simulink model "daqp_block"  (Simulink 10.3)
settings: Solver=VariableStepAuto  StartTime=0.0  StopTime=10.0  RelTol=1e-3
settings Model: Creator=danar20  LastModifiedBy=danar20
settings SolverCC: AlgebraicLoopSolver=Auto
settings DataIOCC: SaveFormat=Dataset  SignalLoggingSaveFormat=Dataset  ReturnWorkspaceOutputs=on
settings OptimizationCC: ExpressionDepthLimit=128  LifeSpan=auto
settings DebuggingCC: UnderspecifiedInitializationDetection=Simplified  MergeDetectMultiDrivingBlocksExec=error  FcnCallInpInsideContextMsg=error  StateNameClashWarn=none  SFUnexpectedBacktrackingDiag=error  SFNoUnconditionalDefaultTransitionDiag=error  SFExecutionAtInitializationDiag=warning  SFMachineParentedDataDiag=error  ArithmeticOperatorsInVariantConditions=error
settings HardwareCC: ProdBitPerPointer=64  ProdBitPerSizeT=64  ProdBitPerPtrDiffT=64  ProdLargestAtomicFloat=Float  ProdIntDivRoundTo=Zero  ProdEndianess=LittleEndian  ProdWordSize=64  ProdHWDeviceType=Intel->x86-64 (Windows64)
settings ModelReferenceCC: PropagateSignalLabelsOutOfModel=on
settings SFSimCC: SimUseLocalCustomCode=on  CustomCodeUndefinedFunction=FilterOut
settings RTWCC: RTWUseLocalCustomCode=on
settings CodeAppCC: StateflowObjectComments=off
settings GRTTargetCC: TargetLangStandard=C99 (ISO)  CombineOutputUpdateFcns=on  GRTInterface=off
settings ConfigComp: CovMetricSettings=dwe  CovSaveCumulativeToWorkspaceVar=off  CovSaveSingleToWorkspaceVar=off  CovExternalEMLEnable=on

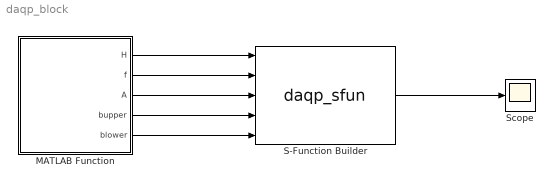
== system daqp_block ==
  MATLAB Function : MATLAB Function  TreatAsAtomicUnit=on
  S-Function Builder : S-Function  FunctionName=daqp_sfun  SFunctionModules=daqp_sfun_wrapper  WizardData=DataTag0  SFunctionDeploymentMode=off  EnableBusSupport=off  mask(S-Function Builder){}
      mask help: Simulink:masks:SFunctionBuilder_MD
      mask init:
      | val = [[.9  0.75 0.75 1 1 .9 .9 1]',[1 1 0.75 0.75 .9 .9 1 .9]'];try , sys = get_param(gcb,'SfunBuilderFcnName');if isempty(sys), sys = get_param(gcb,'FunctionName'); end,catch, sys = get_param(gcb,'FunctionName'); end
      settings: CopyFcn=set_param(gcbh,'LinkStatus','none')  OpenFcn=sfunctionwizard(gcbh)
      mask Display:
      | plot(val(:,1),val(:,2))
      | disp(sys)
      | port_label('input',1,'H')
      | port_label('input',2,'f')
      | port_label('input',3,'A')
      | port_label('input',4,'bupper')
      | port_label('input',5,'blower')
      | port_label('output',1,'u')
  Scope : Scope
  wires:
  MATLAB Function/5(blower) -> S-Function Builder/5
  MATLAB Function/4(bupper) -> S-Function Builder/4
  MATLAB Function/2(f) -> S-Function Builder/2
  MATLAB Function/1(H) -> S-Function Builder/1
  MATLAB Function/3(A) -> S-Function Builder/3
  S-Function Builder/1 -> Scope/1

== matlab function MATLAB Function ==
  data: H output double; f output double; A output double; bupper output double; blower output double
function [H,f,A,bupper,blower] = qp_data()

H = eye(2);
f = [0.5;2];
A = [eye(2); 1 2];
bupper = [1;1;1];
blower = -[1;1;1];
